simulink model "StateFeedback"  (R2020a)
settings: Solver=VariableStepAuto  StartTime=0.0  StopTime=13.0  RelTol=1e-3
undefined symbols (not defined in the file): K1, K2, x1, x2
settings Model: Creator=eyp_d  LastModifiedBy=eyp_d

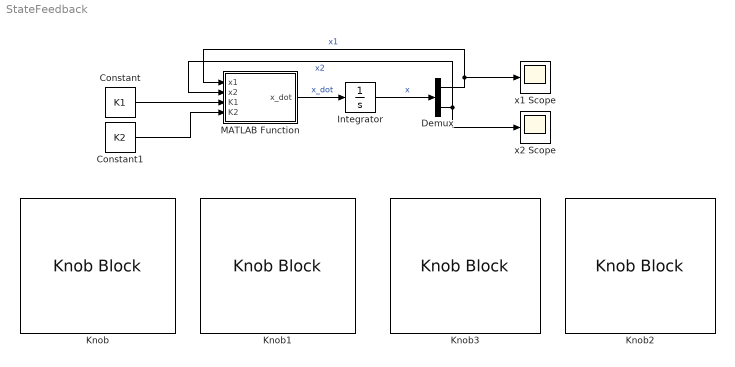
== system StateFeedback ==
  Constant : Constant  Value=K1
  Constant1 : Constant  Value=K2
  Demux : Demux  Outputs=2
  Integrator : Integrator  InitialCondition=[x1, x2]  LowerSaturationLimit=49.27483980109553
  Knob : KnobBlock  ScaleMin=-10  ScaleMax=20
  Knob1 : KnobBlock  ScaleMin=-10  ScaleMax=20
  Knob2 : KnobBlock  ScaleMax=20
  Knob3 : KnobBlock  ScaleMax=20
  MATLAB Function : MATLAB Function  TreatAsAtomicUnit=on
  x1 Scope : Scope
  x2 Scope : Scope
  wires:
  Constant/1 -> MATLAB Function/3(K1)
  Integrator/1 -> Demux/1  "x"
  Demux/2 -> MATLAB Function/2(x2), x2 Scope/1  "x2"
  MATLAB Function/1(x_dot) -> Integrator/1  "x_dot"
  Demux/1 -> x1 Scope/1, MATLAB Function/1(x1)  "x1"
  Constant1/1 -> MATLAB Function/4(K2)

== matlab function StateFeedback/MATLAB Function ==
  data: x1 input; x_dot output; x2 input; K1 input; K2 input
function x_dot = fcn(x1, x2, K1, K2)

A = [0 1; 0 0];
B = [0; 1];
C = [1 0; 0 1];

x = [x1; x2]

A_tilda = A - B *[K1 K2]* C;
x_dot_matrix = A_tilda * x;

x1_dot = x_dot_matrix(1);
x2_dot = x_dot_matrix(2);

x_dot = [x1_dot x2_dot];
